simulink model "Q8"  (R2021b)
settings: Solver=VariableStepAuto  StartTime=0.0  StopTime=50  RelTol=1e-3
values from neighbouring files (symbols this model uses):
  A = [0 0 0 1 0 0 ... (first row only)    [Lab1_code.m]
  B = [0 0 0 ... (first row only)    [Lab1_code.m]
  C = [1 0 0 0 0 0 ... (first row only)    [Lab1_code.m]
  D = [0 0 0 ... (first row only)    [Lab1_code.m]
  x_bias = (-200*5000)/(sqrt(200^2 + 200^2 + 100^2)*m)    [Lab1_code.m]
  y_bias = (-200*5000)/(sqrt(200^2 + 200^2 + 100^2)*m)    [Lab1_code.m]
  z_bias = (-100*5000)/(sqrt(200^2 + 200^2 + 100^2)*m)    [Lab1_code.m]
settings Model: Creator=DSDLn  LastModifiedBy=DSDLn

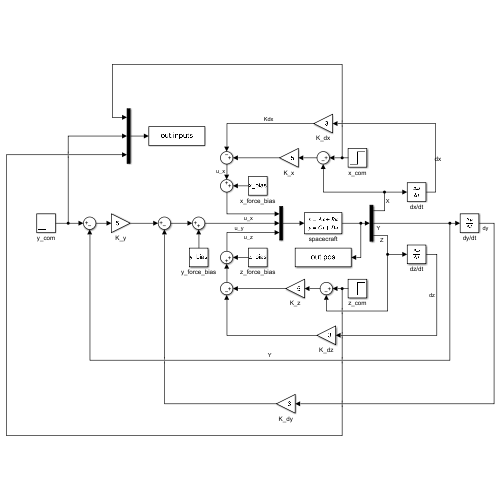
[thumbnail: Simulink's stored preview of the top-level diagram]
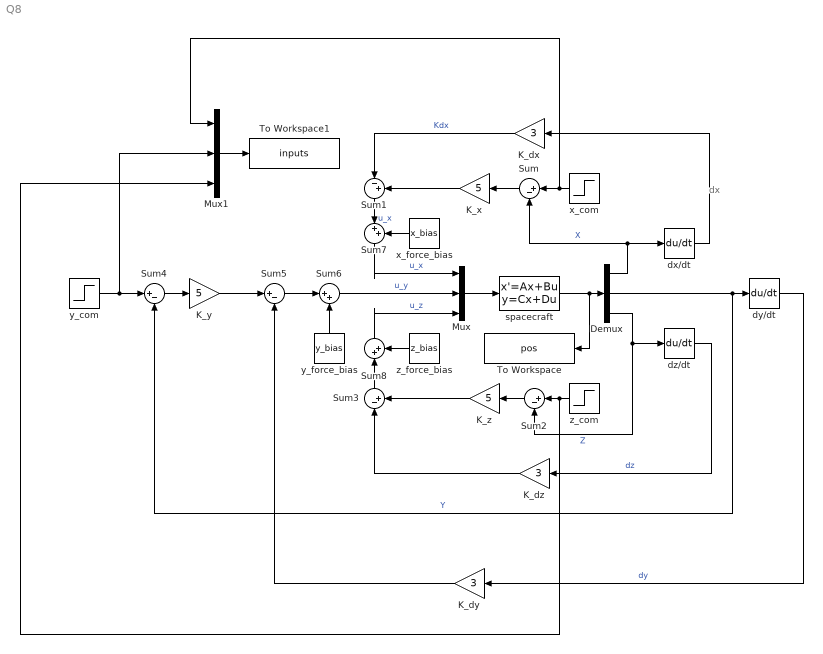
== system Q8 ==
  note: dx
  Demux : Demux  Outputs=3
  K_dx : Gain  Gain=3
  K_dy : Gain  Gain=3
  K_dz : Gain  Gain=3
  K_x : Gain  Gain=5
  K_y : Gain  Gain=5
  K_z : Gain  Gain=5
  Mux : Mux  Inputs=3
  Mux1 : Mux  Inputs=3
  Sum{,2,4..5} (4 alike) : Sum  Inputs=|+-
  Sum1 : Sum  Inputs=|-+
  Sum3 : Sum  Inputs=|-+
  Sum6 : Sum  Inputs=|++
  Sum7 : Sum  Inputs=|++
  Sum8 : Sum  Inputs=|++
  To Workspace : ToWorkspace  VariableName=pos  SampleTime=-1
  To Workspace1 : ToWorkspace  VariableName=inputs  SampleTime=-1
  dx/dt : Derivative
  dy/dt : Derivative
  dz/dt : Derivative
  spacecraft : StateSpace  A=A  B=B  C=C  D=D  InitialCondition=0
  x_com : Step  Time=0  After=5  SampleTime=0.1
  x_force_bias : Constant  Value=x_bias
  y_com : Step  Time=0  SampleTime=0.1
  y_force_bias : Constant  Value=y_bias
  z_com : Step  Time=0  After=4  SampleTime=0.1
  z_force_bias : Constant  Value=z_bias
  wires:
  spacecraft/1 -> To Workspace/1, Demux/1
  Mux/1 -> spacecraft/1
  Demux/1 -> Sum/2, dx/dt/1  "X"
  Demux/2 -> dy/dt/1, Sum4/2  "Y"
  Demux/3 -> dz/dt/1, Sum2/2  "Z"
  x_com/1 -> Sum/1, Mux1/1
  Sum/1 -> K_x/1
  dx/dt/1 -> K_dx/1
  K_x/1 -> Sum1/2
  K_dx/1 -> Sum1/1  "Kdx"
  z_com/1 -> Mux1/3, Sum2/1
  Sum2/1 -> K_z/1
  K_z/1 -> Sum3/2
  K_dz/1 -> Sum3/1
  dz/dt/1 -> K_dz/1  "dz"
  y_com/1 -> Mux1/2, Sum4/1
  Sum4/1 -> K_y/1
  Sum5/1 -> Sum6/1
  dy/dt/1 -> K_dy/1  "dy"
  K_y/1 -> Sum5/1
  K_dy/1 -> Sum5/2
  Sum6/1 -> Mux/2  "u_y"
  y_force_bias/1 -> Sum6/2
  x_force_bias/1 -> Sum7/2
  Sum1/1 -> Sum7/1  "u_x"
  Sum7/1 -> Mux/1  "u_x"
  z_force_bias/1 -> Sum8/2
  Sum3/1 -> Sum8/1
  Sum8/1 -> Mux/3  "u_z"
  Mux1/1 -> To Workspace1/1
